simulink model "MPPT_PSOGSA"  (R2022a)
settings: Solver=FixedStepAuto  StartTime=0.0  StopTime=10  FixedStep=1e-5  RelTol=1e-3
libraries: spsSeriesRLCBranchLib x4, spsDiodeLib x2, spsCurrentMeasurementLib x1, spsMosfetLib x1, spsPVArrayLib x1, spsPWMGeneratorDCDCLib x1, spsVoltageMeasurementLib x1, spspowerguiLib x1
settings Model: Creator=ACER  LastModifiedBy=Thanh Quang
settings DataIOCC: ReturnWorkspaceOutputs=off
settings DebuggingCC: UnconnectedInputMsg=warning  UnconnectedOutputMsg=warning  UnconnectedLineMsg=warning  PregeneratedLibrarySubsystemCodeDiagnostic=none  SFMachineParentedDataDiag=warning  ArithmeticOperatorsInVariantConditions=warning
settings SFSimCC: SimUseLocalCustomCode=off  CustomCodeUndefinedFunction=UseInterfaceOnly
settings RTWCC: RTWUseLocalCustomCode=off

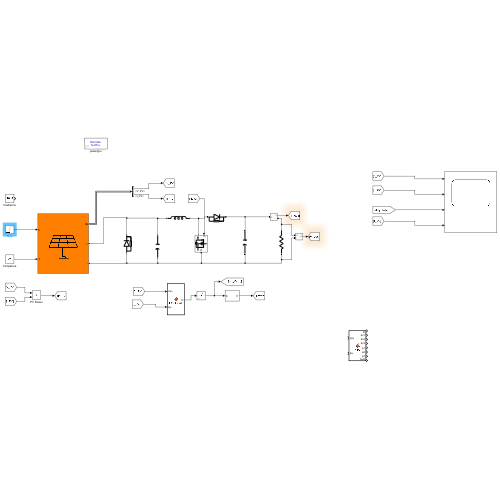
[thumbnail: Simulink's stored preview of the top-level diagram]
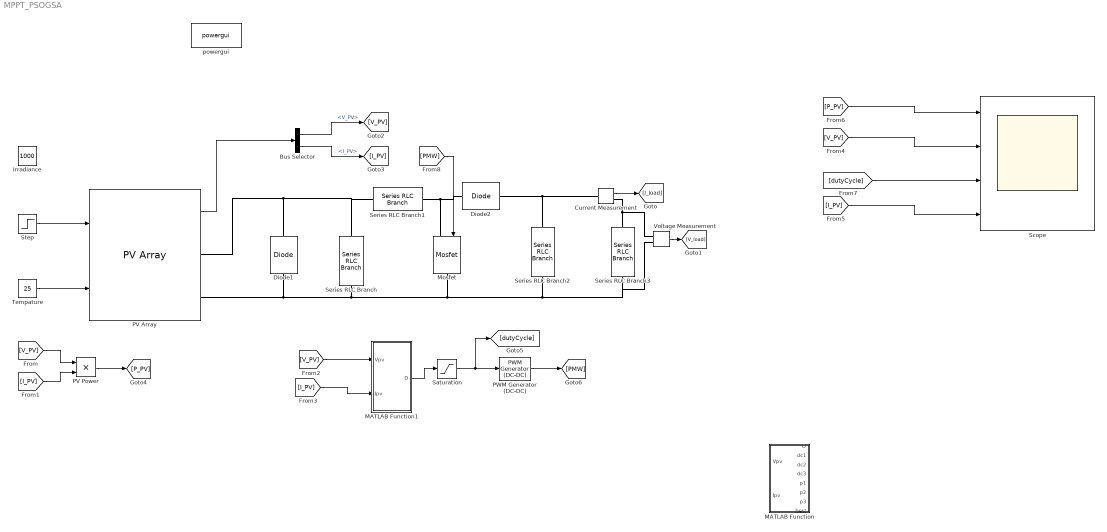
== system MPPT_PSOGSA ==
  Bus Selector : BusSelector  OutputSignals=V_PV,I_PV
  Current Measurement : spsCurrentMeasurementLib/Current Measurement  PhasorSimulation=off  OutputType=Complex  PSBequivalent=0
  Diode1 : spsDiodeLib/Diode  Ron=0.001  Lon=0  Vf=0.8  IC=0  UseSnubber=0  Rs=500  Cs=250e-9  Measurements=off
  Diode2 : spsDiodeLib/Diode  Ron=0.001  Lon=0  Vf=0.8  IC=0  UseSnubber=0  Rs=500  Cs=250e-9  Measurements=off
  Irradiance : Constant  Value=1000  SampleTime=1e-5
  MATLAB Function : MATLAB Function  TreatAsAtomicUnit=on
  MATLAB Function1 : MATLAB Function  TreatAsAtomicUnit=on
  Mosfet : spsMosfetLib/Mosfet  Ron=1e-3  Lon=0  Rd=1e-3  Vfd=0  IC=0  Rs=inf  Cs=inf  Measurements=off
  PV Array : spsPVArrayLib/PV Array  Npar=1  Nser=1  PlotType=array @ 25 deg.C & specified irradiances  S_vec="[ 1000  400 ]"  Temp_C_vec="[ 45 25  ]"  ModuleName=User-defined  PlotWhenSelected=off  Pm=248.977  Ncell=60  Voc=38.4  Isc=8.85  Vm=30.7  Im=8.11  beta_Voc_pc=-0.35599  alpha_Isc_pc=0.07  beta_Voc=-0.1367  alpha_Isc=0.006195  IL=8.8816  I0=2.622e-10  nI=1.0292  Rsh=104.8955  Rs=0.37421  RobustModel=off  RobustCellTemperature=313.3991  BAL=off  Tc=1e-6  Tfilter=1e-5
  PV Power : Product
  PWM Generator (DC-DC) : spsPWMGeneratorDCDCLib/PWM Generator (DC-DC)  Fsw=10000  Ts=1e-5
  Saturation : Saturate  UpperLimit=1  LowerLimit=0
  Scope : Scope  NumInputPorts=4
  Series RLC Branch : spsSeriesRLCBranchLib/Series RLC Branch  LConnTagsString=__new0  RConnTagsString=__new0  BranchType=C  Resistance=1  Inductance=1e-3  SetiL0=off  InitialCurrent=0  Capacitance=5e-3  Setx0=off  InitialVoltage=0  Measurements=None
  Series RLC Branch1 : spsSeriesRLCBranchLib/Series RLC Branch  LConnTagsString=__new0  RConnTagsString=__new0  BranchType=L  Resistance=1  Inductance=2.5e-3  SetiL0=off  InitialCurrent=0  Capacitance=1e-3  Setx0=off  InitialVoltage=0  Measurements=None
  Series RLC Branch2 : spsSeriesRLCBranchLib/Series RLC Branch  LConnTagsString=__new0  RConnTagsString=__new0  BranchType=C  Resistance=1  Inductance=1e-3  SetiL0=off  InitialCurrent=0  Capacitance=250e-6  Setx0=off  InitialVoltage=0  Measurements=None
  Series RLC Branch3 : spsSeriesRLCBranchLib/Series RLC Branch  LConnTagsString=__new0  RConnTagsString=__new0  BranchType=R  Resistance=30  Inductance=1e-3  SetiL0=off  InitialCurrent=0  Capacitance=1e-3  Setx0=off  InitialVoltage=0  Measurements=None
  Step : Step  Time=4  Before=400  After=1000  SampleTime=0
  Tempature : Constant  Value=25
  Voltage Measurement : spsVoltageMeasurementLib/Voltage Measurement  PhasorSimulation=off  OutputType=Complex  PSBequivalent=0
  powergui : spspowerguiLib/powergui  Priority=1  SimulationMode=Discrete  SampleTime=1e-5  frequency=60  Iterations=50  frequencyindice=0  Pbase=100e6  ErrMax=1e-4  UnitsV=kV  UnitsW=MW  buscounter=0  FunctionMessages=off  echomessages=off  EnableUseOfTLC=off  CurrentSourceSwitches=off  DisableSnubberDevices=off  DisableRonSwitches=off  DisableVfSwitches=off  DisplayEquations=off  AutomaticDiscreteSolvers=off  SolverType=Tustin/Backward Euler (TBE)  Interpol=off  ExternalGateDelay=off  methode=off  Ts=100  x0status=blocks  SPID=on  SwTol=0  HookPort=off  NonlinearTolerance=0  nMaxIteration=15  ContinueOnMaxIteration=off  RestoreLinks=warning  ResistiveCurrentMeasurement=off  Frange=[0:2:500]  Ylog=off  Xlog=on  ShowGrid=off  save=off  variable=ZData  structure=0  ZoomFFT=off  StartTime=0.0  cycles=1  DisplayStyle=1  fundamental=60  FreqAxis=off  MaxFrequency=1000  frequencyindicesteady=1  RmsSteady=1  display=off
  wires:
  Tempature/1 -> PV Array/2
  Current Measurement/1 -> [I_load]
  Voltage Measurement/1 -> [V_load]
  PV Array/1 -> Bus Selector/1
  Bus Selector/1 -> [V_PV]  "<V_PV>"
  Bus Selector/2 -> [I_PV]  "<I_PV>"
  [I_PV] -> PV Power/2
  [V_PV] -> PV Power/1
  PV Power/1 -> [P_PV]
  [V_PV] -> MATLAB Function1/1(Vpv)
  [I_PV] -> MATLAB Function1/2(Ipv)
  Saturation/1 -> [dutyCycle], PWM Generator (DC-DC)/1
  PWM Generator (DC-DC)/1 -> [PMW]
  [V_PV] -> Scope/2
  [P_PV] -> Scope/1
  [dutyCycle] -> Scope/3
  [I_PV] -> Scope/4
  [PMW] -> Mosfet/1
  MATLAB Function1/1(D) -> Saturation/1
  Step/1 -> PV Array/1
  connections:
  PV Array/RConn1 -- Diode1/RConn1 -- Series RLC Branch/LConn1 -- Series RLC Branch1/LConn1
  PV Array/RConn2 -- Diode1/LConn1 -- Series RLC Branch/RConn1 -- Voltage Measurement/LConn2 -- Series RLC Branch3/RConn1 -- Series RLC Branch2/RConn1 -- Mosfet/RConn1
  Diode2/LConn1 -- Series RLC Branch1/RConn1 -- Mosfet/LConn1
  Diode2/RConn1 -- Current Measurement/LConn1 -- Series RLC Branch2/LConn1
  Current Measurement/RConn1 -- Voltage Measurement/LConn1 -- Series RLC Branch3/LConn1

== matlab function MPPT_PSOGSA/MATLAB Function1 ==
  settings: updateMethod=DISCRETE
  data: Vpv input; D output; Ipv input
function D = PSOGSA2(Vpv,Ipv)
    %%CHECKED TESTING%%
    persistent u;%u-th particle
    persistent dcurrent;%store current duty cycle
    persistent pbest;%store local best dc for power
    persistent force; %store force
    persistent acceleration; %store acceleration
    persistent mass; % mass
    persistent q; %  strength of mass
    persistent p; %  power for each particle
    persistent p_current; %  power current for each particle
    persistent p_min; %  power min for each particle
    persistent worse;   %store best worse of each particle 
    persistent dc; %store duty cycle ~ position 
    persistent v;  %velocity
    persistent counter; %delay iteration
    persistent gbest;%store global best dc for power
    persistent convergence;%check dc convergence status
    persistent P_prev;%store previous power
    %initialization
    num_agency = 3;
    if(isempty(counter))
        counter = 0;
        dcurrent = 0.5; 
        gbest = 0.5;
        pbest = zeros(num_agency,1);
        worse = zeros(num_agency,1);
        v = zeros (num_agency,1);
        force = zeros(num_agency,1);
        mass = zeros(num_agency,1);
        q = zeros(num_agency,1);
        p = zeros(num_agency,1);
        p_current = zeros(num_agency,1);
        p_min=zeros(num_agency,1);
        p_min(1)= Vpv*Ipv;
        p_min(2)= Vpv*Ipv;
        p_min(3)= Vpv*Ipv;
        acceleration=zeros(num_agency,1);
        u = 0;
        dc = zeros (num_agency,1); 
        P_prev = Ipv*Vpv;
        convergence = 0;

        %initialize position for each particle
        dc(1) = 0.2;
        dc(2) = 0.6;
        dc(3) = 0.9;
    end

    if(convergence == 1)
            if(abs(Vpv*Ipv-P_prev) >= 0.3*P_prev)
                disp("help")
                counter = 0;
                dcurrent = 0.5; 
                gbest = 0.5;
                pbest = zeros(num_agency,1);
                worse = zeros(num_agency,1);
                v = zeros (num_agency,1);
                force = zeros(num_agency,1);
                mass = zeros(num_agency,1);
                q = zeros(num_agency,1);
                p = zeros(num_agency,1);
                p_current = zeros(num_agency,1);
                p_min=zeros(num_agency,1);
                p_min(1)= Vpv*Ipv;
                p_min(2)= Vpv*Ipv;
                p_min(3)= Vpv*Ipv;
                acceleration=zeros(num_agency,1);
                u = 0;
                dc = zeros (num_agency,1); 
                P_prev = Ipv*Vpv;
                convergence = 0;

                %initialize position for each particle
                dc(1) = 0.2;
                dc(2) = 0.6;
                dc(3) = 0.9;
            end
    end
    %Delay for more visualization
    if(counter >=1 && counter < 500)
        D=dcurrent;
        counter= counter+1;
        return;
    end

    if(u>=1 && u<=num_agency)
        p_current(u) = Vpv*Ipv;
        if((Vpv*Ipv)>=p(u))
            p(u) = Vpv*Ipv;
            pbest(u)=dcurrent;
        end
        if(Vpv*Ipv < p_min(u))
            p_min(u) = Vpv*Ipv;
            worse(u) = dcurrent;
        end
    end
    u=u+1;
    if(u== num_agency + 2)
        u=1;
    end
    if(u >= 1 && u <= num_agency)
        D=dc(u);
        dcurrent=D;
        counter=1;
        return;
    elseif(u==num_agency+1)
       
        [~,i]=max(p);
        gbest=pbest(i);
        D=gbest;
        dcurrent=D;
        counter=1;
        %Calculate strength of mass
        disp('chia 1');
        for i = 1:num_agency
            q(i) = (p_current(i) - 0.99*worse(i))/(pbest(i)-worse(i)+ 0.0001);
        end
         %Calculate sum of strength of mass

        sum_strength_of_mass = q(1) + q(2) + q(3);

        %Calculate mass   
        disp('chia 2');
        for i = 1:num_agency
            mass(i) = q(i)*5/sum_strength_of_mass;
        end
        %Calculate force
        G = 6.67430 * 10^-13; %gravitational constant
        e = 2.2204*10^-16;
        disp('chia 3');
        force(1) = rand()*G*(mass(3)*mass(1)*(dc(3)-dc(1))/(Euclidian_distance(dc(3),dc(1))+e) + mass(2)*mass(1)*(dc(3)-dc(1))/(Euclidian_distance(dc(3),dc(1))+e));
        force(2) = rand()*G*(mass(3)*mass(2)*(dc(3)-dc(2))/(Euclidian_distance(dc(3),dc(2))+e) + mass(1)*mass(2)*(dc(1)-dc(2))/(Euclidian_distance(dc(1),dc(2))+e));
        force(3) = rand()*G*(mass(2)*mass(3)*(dc(2)-dc(3))/(Euclidian_distance(dc(2),dc(3))+e) + mass(1)*mass(3)*(dc(1)-dc(3))/(Euclidian_distance(dc(1),dc(3))+e));
        %Calculate acceleration 
        disp('chia 4');
        for i = 1:num_agency
            acceleration(i) = force(i)/mass(i);
        end

        disp('chia 5');
        for i=1:num_agency
            v(i)=updatevelocity(v(i),acceleration(i),dc(i),gbest);
            dc(i)=updateduty(dc(i),v(i));
        end  
        %disp(P_prev)
        %disp(convergence)

        P_prev = Ipv*Vpv;
        convergence = checkconvergence(dc(1),dc(2),dc(3));
        return;

    else
        D=0.5;
    end
end

function status = checkconvergence(d1,d2,d3)
    status = 0;
    rate = 0.002;
    if(abs(d1-d2) < rate)
        if(abs(d1-d3) < rate)
            if(abs(d2-d3) < rate)
                status = 1;
            end
        end
    end
end
function vfinal=updatevelocity(velocity,acceleration,d,gwbest)
    w=0.1;
    c1=1.2;
    c2=1.5;

    vfinal = w*velocity + (rand(1)*c1*(acceleration))+(c2*rand(1)*(gwbest-d));
end
function d = Euclidian_distance(d1,d2)
    d = sqrt(d1^2+d2^2);
end
function dfinal=updateduty(d,velocity)
    dup=d+velocity;
    if(dup>1)
        dfinal=1;
    elseif(dup<0.1)
        dfinal=0.1;
    else
        dfinal=dup;
    end
end

== matlab function MPPT_PSOGSA/MATLAB Function ==
  settings: updateMethod=DISCRETE
  data: Vpv input; D output; Ipv input; dc1 output; dc2 output; dc3 output; p1 output; p2 output; p3 output; best output
function [D, dc1, dc2, dc3, p1, p2, p3, best]  = PSO(Vpv,Ipv)
coder.extrinsic('randi');
persistent u;
persistent dcurrent;
persistent pbest;
persistent p;  %power
persistent dc; %duty cycle
persistent v;  % velocity
persistent counter;
persistent gbest;
persistent Pbest;
persistent Pprev;
%initialization

P = Vpv * Ipv;
if(isempty(counter))
    counter = 0;
    dcurrent = 0.9; %current duty cycle
    gbest = 0.9;
    p = zeros(3,1); %power
    v = zeros (3,1); %voltage
    pbest = zeros(3,1);
    u = 0;
    dc = zeros (3,1); %duty cycle
    Pprev = 0;
    Pbest = 0;
    %initial dc for each particle
    dc(1)=randi( [5 330])/1000;
        dc(2)=randi( [330 660])/1000;
        dc(3)=randi( [660 995])/1000;
end

if (P > Pbest)
    Pbest = P;
end

%At the first time, this if ignored (counter = 0)
%Delay

dc1 = dc(1);
dc2 = dc(2);
dc3 = dc(3);
p1 = p(1);
p2 = p(2);
p3 = p(3);
best = Pbest;
if(counter >= 1 && counter < 100)
    D = dcurrent;
    counter = counter + 1;
    return;
end
counter = 0; %reset the counter


if abs(P-Pprev) < 0.1
    if abs (P - Pbest) < 20
    counter = 0;
    dcurrent = 0.3; %current duty cycle
    gbest = 0.3;
    p = zeros(3,1); %power
    v = zeros (3,1); %voltage
    pbest = zeros(3,1);
    u = 0;
    dc = zeros (3,1); %duty cycle
    %initial dc for each particle
    dc(1)=randi( [5 330])/1000;
    dc(2)=randi( [330 660])/1000;
    dc(3)=randi( [660 995])/1000;
    end
end

Pprev = P;

%calculate fittnes function (power) of each particle
%then compare the fitness, if better then update
if(u>=1 && u<=3)
    if((Vpv*Ipv) > p(u))
        p(u) = Vpv*Ipv;
        pbest(u) = dcurrent;
    end
end

u=u+1;
%At the first time, this is executed because it consist the condition
%u==0 (initial value of u)
if(u==5)
    u=1;
end

if(u==1)
    D=dc(u);
    dcurrent=D;
    counter=1;
    return;
elseif(u==2)
    D=dc(u);
    dcurrent=D;
    counter=1;
    return;
elseif(u==3)
    D=dc(u);
    dcurrent=D;
    counter=1;
    return;
elseif(u==4)
    [m,i] = max(p); %find the indices of the maximum values of P (max power) and returns them in output vector i
    gbest = pbest(i); %find the location(duty) of the particle which has max P
    D = gbest;
    dcurrent = D;
    counter = 1;
    %update velocity and duty cycle
    v(1) = updatevelocity(v(1),pbest(1),dc(1),gbest);
    v(2) = updatevelocity(v(2),pbest(2),dc(2),gbest);
    v(3) = updatevelocity(v(3),pbest(3),dc(3),gbest);
    
    %update duty cycle
    dc(1) = updateduty(dc(1),v(1));
    dc(2) = updateduty(dc(2),v(2));
    dc(3) = updateduty(dc(3),v(3));
    
    
    return;
    
 
else
    
    D=rand;
end

end 

function vfinal = updatevelocity(velocity,pobest,d,gwbest)
% PSO parameters
w = 0.1;
c1 = 1.2;
c2 = 1.2;
vfinal = (w*velocity) + (c1*rand(1)*(pobest-d))+(c2*rand(1)*(gwbest-d));
end

function dfinal = updateduty(d,velocity)
dup = d+velocity;
if(dup > 1)
    dfinal = 1;
elseif(dup < 0)
    dfinal = 0;
else
    dfinal = dup;
end
end
